simulink model "towing_project"  (Simulink 10.1)
settings: Solver=ode4  StartTime=0.0  StopTime=1000  FixedStep=1  RelTol=1e-3  EnableMultiTasking=on
PreLoadFcn:
  | load('Initialization_data.mat');
undefined symbols (not defined in the file): D1, M1, Ma1, magnitude, p00, p10, p20, p30, p40
libraries: simulink x8, simulink_extras x4
(part 2 of 2)

== system towing_project/local DP4/Tug/[-inf inf] to [-pi pi]1 ==
  note: x
  note: r
  x [-inf inf] : Inport
  Constant : Constant  Value=2*pi
  Gain : Gain  Gain=pi  SaturateOnIntegerOverflow=on  OutDataTypeStr=Inherit: Same as input  ParamDataTypeStr=Inherit: Same as input
  Math Function : Math  Operator=rem  SignedPower=on  SaturateOnIntegerOverflow=on
  Saturation : Saturate  UpperLimit=1e10  LowerLimit=-1e10
  Sign : Signum
  Sum : Sum  Inputs=|+-  SaturateOnIntegerOverflow=on
  Sum1 : Sum  Inputs=|++  SaturateOnIntegerOverflow=on
  y [-pi pi] : Outport
  wires:
  x [-inf inf]/1 -> Saturation/1
  Sign/1 -> Gain/1
  Gain/1 -> Sum/2, Sum1/2
  Sum1/1 -> Math Function/1
  Constant/1 -> Math Function/2
  Math Function/1 -> Sum/1
  Sum/1 -> y [-pi pi]/1
  Saturation/1 -> Sum1/1, Sign/1

== system towing_project/local DP4/Tug DP controller/Transposed rotation  matrix in yaw ==
  psi : Inport
  V : Inport  Port=2
  Mux : Mux  Inputs=2
  Mux1 : Mux  Inputs=3
  Row1 : Fcn  Expr=cos(u(1))*u(2)+sin(u(1))*u(3)
  Row2 : Fcn  Expr=-sin(u(1))*u(2)+cos(u(1))*u(3)
  Row3 : Fcn  Expr=u(4)
  Out1 : Outport
  wires:
  Mux/1 -> Row3/1, Row2/1, Row1/1
  Row1/1 -> Mux1/1
  Row2/1 -> Mux1/2
  Row3/1 -> Mux1/3
  Mux1/1 -> Out1/1
  psi/1 -> Mux/1
  V/1 -> Mux/2

== system towing_project/local DP4/Tug DP controller/[-inf inf] to [-pi pi]1 ==
  note: x
  note: r
  x [-inf inf] : Inport
  Constant : Constant  Value=2*pi
  Gain : Gain  Gain=pi  SaturateOnIntegerOverflow=on  OutDataTypeStr=Inherit: Same as input  ParamDataTypeStr=Inherit: Same as input
  Math Function : Math  Operator=rem  SignedPower=on  SaturateOnIntegerOverflow=on
  Saturation : Saturate  UpperLimit=1e10  LowerLimit=-1e10
  Sign : Signum
  Sum : Sum  Inputs=|+-  SaturateOnIntegerOverflow=on
  Sum1 : Sum  Inputs=|++  SaturateOnIntegerOverflow=on
  y [-pi pi] : Outport
  wires:
  x [-inf inf]/1 -> Saturation/1
  Sign/1 -> Gain/1
  Gain/1 -> Sum/2, Sum1/2
  Sum1/1 -> Math Function/1
  Constant/1 -> Math Function/2
  Math Function/1 -> Sum/1
  Sum/1 -> y [-pi pi]/1
  Saturation/1 -> Sum1/1, Sign/1

== system towing_project/local DP4/Tug DP controller/[-inf inf] to [-pi pi]2 ==
  note: r
  note: x
  x [-inf inf] : Inport
  Constant : Constant  Value=2*pi
  Gain : Gain  Gain=pi  SaturateOnIntegerOverflow=on  OutDataTypeStr=Inherit: Same as input  ParamDataTypeStr=Inherit: Same as input
  Math Function : Math  Operator=rem  SignedPower=on  SaturateOnIntegerOverflow=on
  Saturation : Saturate  UpperLimit=1e10  LowerLimit=-1e10
  Sign : Signum
  Sum : Sum  Inputs=|+-  SaturateOnIntegerOverflow=on
  Sum1 : Sum  Inputs=|++  SaturateOnIntegerOverflow=on
  y [-pi pi] : Outport
  wires:
  Saturation/1 -> Sign/1, Sum1/1
  Sum/1 -> y [-pi pi]/1
  Math Function/1 -> Sum/1
  Constant/1 -> Math Function/2
  Sum1/1 -> Math Function/1
  Gain/1 -> Sum1/2, Sum/2
  Sign/1 -> Gain/1
  x [-inf inf]/1 -> Saturation/1

== system towing_project/local DP1/Tug/Coriolis and centripetal forces/Subsystem ==
  v : Inport
  r : Inport  Port=2
  -a22 : Gain  Gain=-M1(2,2)-Ma1(2,2)  Multiplication=Matrix(K*u)  SaturateOnIntegerOverflow=on  OutDataTypeStr=Inherit: Same as input  ParamDataTypeStr=Inherit: Same as input
  -a26 : Gain  Gain=-M1(2,3)-Ma1(2,3)  Multiplication=Matrix(K*u)  SaturateOnIntegerOverflow=on  OutDataTypeStr=Inherit: Same as input  ParamDataTypeStr=Inherit: Same as input
  Add : Sum
  Math Function : Math  Operator=magnitude^2  SignedPower=on  SaturateOnIntegerOverflow=on
  Product : Product  RndMeth=Zero
  x direction : Outport
  wires:
  v/1 -> Product/1
  r/1 -> Product/2, Math Function/1
  Product/1 -> -a22/1
  Math Function/1 -> -a26/1
  -a22/1 -> Add/1
  -a26/1 -> Add/2
  Add/1 -> x direction/1

== system towing_project/local DP1/Tug/Coriolis and centripetal forces/Subsystem1 ==
  u : Inport
  r : Inport  Port=2
  Product : Product  RndMeth=Zero
  a11 : Gain  Gain=M1(1,1)+Ma1(1,1)  Multiplication=Matrix(K*u)  SaturateOnIntegerOverflow=on  OutDataTypeStr=Inherit: Same as input  ParamDataTypeStr=Inherit: Same as input
  y direction : Outport
  wires:
  Product/1 -> a11/1
  r/1 -> Product/2
  u/1 -> Product/1
  a11/1 -> y direction/1

== system towing_project/local DP1/Tug/Coriolis and centripetal forces/Subsystem2 ==
  u : Inport
  v : Inport  Port=2
  r : Inport  Port=3
  Add : Sum
  Add1 : Sum  Inputs=+-
  Product : Product  RndMeth=Zero
  Product1 : Product  RndMeth=Zero
  a11 : Gain  Gain=M1(1,1)+Ma1(1,1)  Multiplication=Matrix(K*u)  SaturateOnIntegerOverflow=on  OutDataTypeStr=Inherit: Same as input  ParamDataTypeStr=Inherit: Same as input
  a22 : Gain  Gain=M1(2,2)+Ma1(2,2)  Multiplication=Matrix(K*u)  SaturateOnIntegerOverflow=on  OutDataTypeStr=Inherit: Same as input  ParamDataTypeStr=Inherit: Same as input
  a62 : Gain  Gain=M1(3,2)+Ma1(3,2)  Multiplication=Matrix(K*u)  SaturateOnIntegerOverflow=on  OutDataTypeStr=Inherit: Same as input  ParamDataTypeStr=Inherit: Same as input
  yaw direction : Outport
  wires:
  u/1 -> Product/1, Product1/1
  r/1 -> Product/2
  Product/1 -> a62/1
  v/1 -> Product1/2
  Product1/1 -> a22/1, a11/1
  a22/1 -> Add1/1
  a11/1 -> Add1/2
  Add1/1 -> Add/2
  a62/1 -> Add/1
  Add/1 -> yaw direction/1

== system towing_project/local DP2/Tug/Coriolis and centripetal forces/Subsystem ==
  v : Inport
  r : Inport  Port=2
  -a22 : Gain  Gain=-M1(2,2)-Ma1(2,2)  Multiplication=Matrix(K*u)  SaturateOnIntegerOverflow=on  OutDataTypeStr=Inherit: Same as input  ParamDataTypeStr=Inherit: Same as input
  -a26 : Gain  Gain=-M1(2,3)-Ma1(2,3)  Multiplication=Matrix(K*u)  SaturateOnIntegerOverflow=on  OutDataTypeStr=Inherit: Same as input  ParamDataTypeStr=Inherit: Same as input
  Add : Sum
  Math Function : Math  Operator=magnitude^2  SignedPower=on  SaturateOnIntegerOverflow=on
  Product : Product  RndMeth=Zero
  x direction : Outport
  wires:
  v/1 -> Product/1
  r/1 -> Product/2, Math Function/1
  Product/1 -> -a22/1
  Math Function/1 -> -a26/1
  -a22/1 -> Add/1
  -a26/1 -> Add/2
  Add/1 -> x direction/1

== system towing_project/local DP2/Tug/Coriolis and centripetal forces/Subsystem1 ==
  u : Inport
  r : Inport  Port=2
  Product : Product  RndMeth=Zero
  a11 : Gain  Gain=M1(1,1)+Ma1(1,1)  Multiplication=Matrix(K*u)  SaturateOnIntegerOverflow=on  OutDataTypeStr=Inherit: Same as input  ParamDataTypeStr=Inherit: Same as input
  y direction : Outport
  wires:
  Product/1 -> a11/1
  r/1 -> Product/2
  u/1 -> Product/1
  a11/1 -> y direction/1

== system towing_project/local DP2/Tug/Coriolis and centripetal forces/Subsystem2 ==
  u : Inport
  v : Inport  Port=2
  r : Inport  Port=3
  Add : Sum
  Add1 : Sum  Inputs=+-
  Product : Product  RndMeth=Zero
  Product1 : Product  RndMeth=Zero
  a11 : Gain  Gain=M1(1,1)+Ma1(1,1)  Multiplication=Matrix(K*u)  SaturateOnIntegerOverflow=on  OutDataTypeStr=Inherit: Same as input  ParamDataTypeStr=Inherit: Same as input
  a22 : Gain  Gain=M1(2,2)+Ma1(2,2)  Multiplication=Matrix(K*u)  SaturateOnIntegerOverflow=on  OutDataTypeStr=Inherit: Same as input  ParamDataTypeStr=Inherit: Same as input
  a62 : Gain  Gain=M1(3,2)+Ma1(3,2)  Multiplication=Matrix(K*u)  SaturateOnIntegerOverflow=on  OutDataTypeStr=Inherit: Same as input  ParamDataTypeStr=Inherit: Same as input
  yaw direction : Outport
  wires:
  u/1 -> Product/1, Product1/1
  r/1 -> Product/2
  Product/1 -> a62/1
  v/1 -> Product1/2
  Product1/1 -> a22/1, a11/1
  a22/1 -> Add1/1
  a11/1 -> Add1/2
  Add1/1 -> Add/2
  a62/1 -> Add/1
  Add/1 -> yaw direction/1

== system towing_project/local DP3/Tug/Coriolis and centripetal forces/Subsystem ==
  v : Inport
  r : Inport  Port=2
  -a22 : Gain  Gain=-M1(2,2)-Ma1(2,2)  Multiplication=Matrix(K*u)  SaturateOnIntegerOverflow=on  OutDataTypeStr=Inherit: Same as input  ParamDataTypeStr=Inherit: Same as input
  -a26 : Gain  Gain=-M1(2,3)-Ma1(2,3)  Multiplication=Matrix(K*u)  SaturateOnIntegerOverflow=on  OutDataTypeStr=Inherit: Same as input  ParamDataTypeStr=Inherit: Same as input
  Add : Sum
  Math Function : Math  Operator=magnitude^2  SignedPower=on  SaturateOnIntegerOverflow=on
  Product : Product  RndMeth=Zero
  x direction : Outport
  wires:
  v/1 -> Product/1
  r/1 -> Product/2, Math Function/1
  Product/1 -> -a22/1
  Math Function/1 -> -a26/1
  -a22/1 -> Add/1
  -a26/1 -> Add/2
  Add/1 -> x direction/1

== system towing_project/local DP3/Tug/Coriolis and centripetal forces/Subsystem1 ==
  u : Inport
  r : Inport  Port=2
  Product : Product  RndMeth=Zero
  a11 : Gain  Gain=M1(1,1)+Ma1(1,1)  Multiplication=Matrix(K*u)  SaturateOnIntegerOverflow=on  OutDataTypeStr=Inherit: Same as input  ParamDataTypeStr=Inherit: Same as input
  y direction : Outport
  wires:
  Product/1 -> a11/1
  r/1 -> Product/2
  u/1 -> Product/1
  a11/1 -> y direction/1

== system towing_project/local DP3/Tug/Coriolis and centripetal forces/Subsystem2 ==
  u : Inport
  v : Inport  Port=2
  r : Inport  Port=3
  Add : Sum
  Add1 : Sum  Inputs=+-
  Product : Product  RndMeth=Zero
  Product1 : Product  RndMeth=Zero
  a11 : Gain  Gain=M1(1,1)+Ma1(1,1)  Multiplication=Matrix(K*u)  SaturateOnIntegerOverflow=on  OutDataTypeStr=Inherit: Same as input  ParamDataTypeStr=Inherit: Same as input
  a22 : Gain  Gain=M1(2,2)+Ma1(2,2)  Multiplication=Matrix(K*u)  SaturateOnIntegerOverflow=on  OutDataTypeStr=Inherit: Same as input  ParamDataTypeStr=Inherit: Same as input
  a62 : Gain  Gain=M1(3,2)+Ma1(3,2)  Multiplication=Matrix(K*u)  SaturateOnIntegerOverflow=on  OutDataTypeStr=Inherit: Same as input  ParamDataTypeStr=Inherit: Same as input
  yaw direction : Outport
  wires:
  u/1 -> Product/1, Product1/1
  r/1 -> Product/2
  Product/1 -> a62/1
  v/1 -> Product1/2
  Product1/1 -> a22/1, a11/1
  a22/1 -> Add1/1
  a11/1 -> Add1/2
  Add1/1 -> Add/2
  a62/1 -> Add/1
  Add/1 -> yaw direction/1

== system towing_project/local DP4/Tug/Coriolis and centripetal forces/Subsystem ==
  v : Inport
  r : Inport  Port=2
  -a22 : Gain  Gain=-M1(2,2)-Ma1(2,2)  Multiplication=Matrix(K*u)  SaturateOnIntegerOverflow=on  OutDataTypeStr=Inherit: Same as input  ParamDataTypeStr=Inherit: Same as input
  -a26 : Gain  Gain=-M1(2,3)-Ma1(2,3)  Multiplication=Matrix(K*u)  SaturateOnIntegerOverflow=on  OutDataTypeStr=Inherit: Same as input  ParamDataTypeStr=Inherit: Same as input
  Add : Sum
  Math Function : Math  Operator=magnitude^2  SignedPower=on  SaturateOnIntegerOverflow=on
  Product : Product  RndMeth=Zero
  x direction : Outport
  wires:
  v/1 -> Product/1
  r/1 -> Product/2, Math Function/1
  Product/1 -> -a22/1
  Math Function/1 -> -a26/1
  -a22/1 -> Add/1
  -a26/1 -> Add/2
  Add/1 -> x direction/1

== system towing_project/local DP4/Tug/Coriolis and centripetal forces/Subsystem1 ==
  u : Inport
  r : Inport  Port=2
  Product : Product  RndMeth=Zero
  a11 : Gain  Gain=M1(1,1)+Ma1(1,1)  Multiplication=Matrix(K*u)  SaturateOnIntegerOverflow=on  OutDataTypeStr=Inherit: Same as input  ParamDataTypeStr=Inherit: Same as input
  y direction : Outport
  wires:
  Product/1 -> a11/1
  r/1 -> Product/2
  u/1 -> Product/1
  a11/1 -> y direction/1

== system towing_project/local DP4/Tug/Coriolis and centripetal forces/Subsystem2 ==
  u : Inport
  v : Inport  Port=2
  r : Inport  Port=3
  Add : Sum
  Add1 : Sum  Inputs=+-
  Product : Product  RndMeth=Zero
  Product1 : Product  RndMeth=Zero
  a11 : Gain  Gain=M1(1,1)+Ma1(1,1)  Multiplication=Matrix(K*u)  SaturateOnIntegerOverflow=on  OutDataTypeStr=Inherit: Same as input  ParamDataTypeStr=Inherit: Same as input
  a22 : Gain  Gain=M1(2,2)+Ma1(2,2)  Multiplication=Matrix(K*u)  SaturateOnIntegerOverflow=on  OutDataTypeStr=Inherit: Same as input  ParamDataTypeStr=Inherit: Same as input
  a62 : Gain  Gain=M1(3,2)+Ma1(3,2)  Multiplication=Matrix(K*u)  SaturateOnIntegerOverflow=on  OutDataTypeStr=Inherit: Same as input  ParamDataTypeStr=Inherit: Same as input
  yaw direction : Outport
  wires:
  u/1 -> Product/1, Product1/1
  r/1 -> Product/2
  Product/1 -> a62/1
  v/1 -> Product1/2
  Product1/1 -> a22/1, a11/1
  a22/1 -> Add1/1
  a11/1 -> Add1/2
  Add1/1 -> Add/2
  a62/1 -> Add/1
  Add/1 -> yaw direction/1

== matlab function Consensus Control ==
  data: p0 input double; pd1 output double; v0 input double; state input double; pd2 output double; pd3 output double; pd4 output double
% function [pd1, pd2] = consensus_guidance(p0, v0, p1, v1, p2, v2)
function [pd1, pd2, pd3, pd4] = consensus_guidance(p0, v0, state)
% 默认输入和输出的单位为角度
% % p0, v0的角度单位都是弧度
% p(全局坐标系）， v(局部坐标系）
% dot_p (全局坐标系）
% clear all; clc;
% p1 = [397, 237, 31]';
% p2 = [397, -237, -31]';
% p0 = [1, 0, 0]';
% v0 = zeros(3, 1);
% v1 = zeros(3, 1);
% v2 = zeros(3, 1);

p1 = state(1:3);
v1 = state(4:6);
p2 = state(7:9);
v2 = state(10:12);
p3 = state(13 : 15);
v3 = state(16 : 18);
p4 = state(19 :21);
v4 = state(22 : 24);

% 需要声明lqr函数为外部函数，否则simulink会编译报错
coder.extrinsic('lqr'); 

pd1 = zeros(3, 1);
pd2 = zeros(3, 1);
pd3 = zeros(3, 1);
pd4 = zeros(3, 1);

% 角度单位转化成弧度
deg_to_rad = pi / 180;
p0(3) = p0(3) * deg_to_rad;
p1(3) = p1(3) * deg_to_rad;
p2(3) = p2(3) * deg_to_rad;
p3(3) = p3(3) * deg_to_rad;
p4(3) = p4(3) * deg_to_rad;

dotP0 = v0; % 输入的v0是在大地坐标系下的   
dotP0(3) = dotP0(3) * deg_to_rad;

% % 将角度转化为（-pi, pi)
% p0(3) = transfer_deg(p0(3));
% p1(3) = transfer_deg(p1(3));
% p2(3) = transfer_deg(p2(3));

% dotP0 = V_to_dotP(p0, v0);
dotP1 = V_to_dotP(p1, v1);
dotP2 = V_to_dotP(p2, v2);
dotP3 = V_to_dotP(p3, v3);
dotP4 = V_to_dotP(p4, v4);

% 定义状态变量
x0 = [p0; dotP0];
x1 = [p1; dotP1];
x2 = [p2; dotP2];
x3 = [p3; dotP3];
x4 = [p4; dotP4];

%% 编队的相对位置,这个是在局部坐标系下的，需要转化为大地坐标系下
deta10 = [397, 237, 31 * deg_to_rad, 0, 0, 0]';
deta20 = [397, -237, -31 * deg_to_rad, 0, 0, 0]';
deta30 = [-397, -237, -149 * deg_to_rad, 0, 0, 0]';
deta40 = [-397, 237, 149 * deg_to_rad, 0, 0, 0]';

deta12 = deta10 - deta20;   deta21 = -deta12;
deta14 = deta10 - deta40;   deta41 = -deta14;
deta23 = deta20 - deta30;   deta32 = -deta23;
deta34 = deta30 - deta40;   deta43 = -deta34;


fai0 = p0(3);   fai1 = p1(3);   fai2 = p2(3);
fai3 = p3(3);   fai4 = p4(3);

%拖船到母船的距离
Lc1 = sqrt(deta10(1)^2 + deta10(2)^2);
Lc2 = sqrt(deta20(1)^2 + deta20(2)^2);
Lc3 = sqrt(deta30(1)^2 + deta30(2)^2);
Lc4 = sqrt(deta40(1)^2 + deta40(2)^2);

deta10(1:2) = [cos(fai0), -sin(fai0); sin(fai0), cos(fai0)] * deta10(1:2);
deta20(1:2) = [cos(fai0), -sin(fai0); sin(fai0), cos(fai0)] * deta20(1:2);
deta30(1:2) = [cos(fai0), -sin(fai0); sin(fai0), cos(fai0)] * deta30(1:2);
deta40(1:2) = [cos(fai0), -sin(fai0); sin(fai0), cos(fai0)] * deta40(1:2);

deta12 = deta10 - deta20;   deta21 = -deta12;
deta14 = deta10 - deta40;   deta41 = -deta14;
deta23 = deta20 - deta30;   deta32 = -deta23;
deta34 = deta30 - deta40;   deta43 = -deta34;
% deta12 = deta10 - deta20;
% deta21 = - deta12;



% 先假定aij = 1, gi = 1;， 需要加上相对位置
e1 = x2 - x1 - deta21 + x4 - x1 - deta41 + x0 - x1 + deta10;
e2 = x1 - x2 - deta12 + x3 - x2 - deta32 + x0 - x2 + deta20;
e3 = x2 - x3 - deta23 + x4 - x3 - deta43 + x0 - x3 + deta30;
e4 = x1 - x4 - deta14 + x3 - x4 - deta34 + x0 - x4 + deta40;

e1(3) = transfer_deg(e1(3));
e2(3) = transfer_deg(e2(3));
e3(3) = transfer_deg(e3(3));
e4(3) = transfer_deg(e4(3));

%% 定义状态反馈方程的系数，求解raccati方程
wn = 0.05; 
cd = 0.7;

A1 = -2 * cd * wn * eye(3);
A0 = -wn^2 * eye(3);
B1 = -A0;

A = [zeros(3, 3), eye(3); A0, A1];
B = [zeros(3, 3); B1];

% Q = diag([0.01, 0.01, 4e-8, 100, 100, 4e-4]);
% R = diag([0.01, 0.01, 4e-8]);
Q = 4 * eye(6);
R = 1 * eye(3);
N = [];
[K, S, e] = lqr(A, B, Q, R, N);

K;
u1 = K * e1;
u2 = K * e2;
u3 = K * e3;
u4 = K * e4;

pd1 = u1; 
pd2 = u2;
pd3 = u3; 
pd4 = u4;

pd1 = pd1 + p1;
pd2 = pd2 + p2;
pd3 = pd3 + p3;
pd4 = pd4 + p4;

pd1(3) = transfer_deg(pd1(3));
pd2(3) = transfer_deg(pd2(3));
pd3(3) = transfer_deg(pd3(3));
pd4(3) = transfer_deg(pd4(3));


%% 函数输入输出都是角度
pd1(3) = pd1(3) / 3.14 * 180;
pd2(3) = pd2(3) / 3.14 * 180;
pd3(3) = pd3(3) / 3.14 * 180;
pd4(3) = pd4(3) / 3.14 * 180;

end







%% 旋转矩阵
function R = RotationMatrix(p)
fai = p(3);
R = zeros(3, 3);
R = [cos(fai), -sin(fai), 0;
    sin(fai), cos(fai), 0;
    0, 0, 1];
end

%% 将速度转换成全局坐标系中，即p的微分
function dot_P = V_to_dotP(p, v)
R = zeros(3, 3);
R = RotationMatrix(p);
dot_P = R * v;

end

%% 将角度转化为（-pi, pi)
function y = transfer_deg(x)
    y = -sign(x) * pi + rem((x + sign(x) * pi), 2 * pi);
end
